simulink model "DynamicFFT_Ex2"  (R2024a)
settings: Solver=VariableStepAuto  StartTime=0.0  StopTime=2  RelTol=1e-3
model workspace (MAT data in the model file):
  frame_size = 512
  max_fft_size = 512
undefined symbols (not defined in the file): None, S, vsva2197, xcvc1902
libraries: matrix_library x2, aieDSP x1, dspobslib x1, dspsrcs4 x1, aieUtilities x1, vmcUtilities x1
settings Model: Creator=sdegala  LastModifiedBy=robg
settings ModelReferenceCC: EnableRefExpFcnMdlSchedulingChecks=on
settings RTWCC: GPUComputeCapability=3.5
settings ConfigComp: CovBoundaryAbsTol=1.0e-5

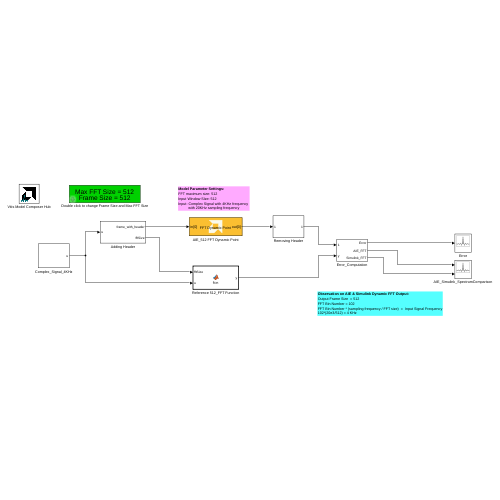
[thumbnail: Simulink's stored preview of the top-level diagram]
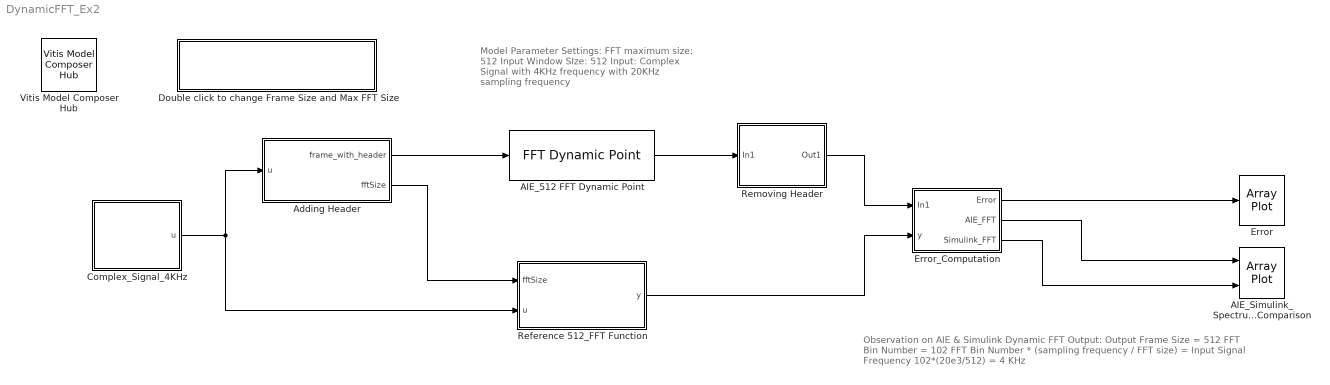
== system DynamicFFT_Ex2 ==
  note: Model Parameter Settings:
      | FFT maximum size: 512
      | Input Window SIze: 512
      | Input: Complex Signal with 4KHz frequency
      | with 20KHz sampling frequency
  note: Observation on AIE & Simulink Dynamic FFT Output:
      | Output Frame Size = 512
      | FFT Bin Number = 102
      | FFT Bin Number * (sampling frequency / FFT size) = Input Signal Frequency
      | 102*(20e3/512) = 4 KHz
  AIE_512 FFT Dynamic Point : aieDSP/FFT Dynamic Point  AIE_VARIANT=1  data_type=cfloat  data_out_type=cfloat  twiddle_type=cfloat  point_size=512  input_window_size=512  shift_val=0  rnd_mode=Round symmetrical to infinity  sat_mode=0-None  ssr=1  twiddle_mode=0  use_ssr_widget_kernels=off  casc_length=1  transform_fft_nifft=1  TP_API=0  TP_DYN_PT_SIZE=1  blockJsonConstraints=[]  blockJsonConstraintsInternal=[]  spec=vmc_dyn_pt_fft.json  SerializedMaskParamNames=[]  SerializedMaskParamValues=[]  SerializedMaskParamVisibilities=[]  block_type=FFT Dynamic Point  SerializedMaskParamDataypes=uint|typename|typename|typename|uint|uint|uint|uint|uint|uint|uint|uint|uint|uint|uint|uint  SerializedMaskParamEnumStrArr=0|0|0|0|0|0|0|Round to positive infinity,Round to negative infinity,Round symmetrical to infinity,Round symmetrical to zero,Round convergent to even,Round convergent to odd|0-None,1-Asymmetric,3-Symmetric|0|0|0|0|0|0|0  SerializedMaskParamEnumValArr=0|0|0|0|0|0|0|2,3,4,5,6,7|0,1,3|0|0|0|0|0|0|0  SerializedMaskParamVectorArr=0|0|0|0|0|0|0|0|0|0|0|0|0|0|0|0  SerializedMaskParamKeys=AIE_VARIANT|TT_DATA|TT_OUT_DATA|TT_TWIDDLE|TP_POINT_SIZE|TP_WINDOW_VSIZE|TP_SHIFT|TP_RND|TP_SAT|TP_PARALLEL_POWER|TP_TWIDDLE_MODE|TP_USE_WIDGETS|TP_CASC_LEN|TP_FFT_NIFFT|TP_API|TP_DYN_PT_SIZE
  AIE_Simulink_SpectrumComparison : ArrayPlot  NumInputPorts=2  WindowPosition=[5.000000,41.000000,1272.000000,651.000000,]  PlotType=Line  AxesScaling=Manual  YLimits=[-100,1100]  ShowLegend=on
  Adding Header : Subsystem
  Complex_Signal_4KHz : Subsystem
  Double click to change Frame Size and Max FFT Size : Subsystem  mask{max_fft_size=512, frame_size=512}
      mask prompts: max_fft_size "Max FFT Size"; frame_size "Frame Size"
      mask help: Set the FFT length
      mask TypeOptions max_fft_size: 128 | 256 | 512 | 1024 | 2048 | 4096
      mask Callback max_fft_size:
      | max_fft_size = str2double(get_param(gcb,'max_fft_size'));
      | hws = get_param(bdroot, 'modelworkspace');
      | hws.assignin('max_fft_size', max_fft_size);
      mask Callback frame_size:
      | frame_size = str2double(get_param(gcb,'frame_size'));
      | hws = get_param(bdroot, 'modelworkspace');
      | hws.assignin('frame_size', frame_size);
      mask Display:
      | max_fft_size = get_param(gcb,'max_fft_size');
      | frame_size = get_param(gcb,'frame_size');
      | 
      | disp(['\fontsize{18}Max FFT Size = ' max_fft_size newline 'Frame Size = ' frame_size], 'texmode', 'on');
  Error : ArrayPlot  WindowPosition=[432.000000,41.000000,845.000000,423.000000,]  PlotType=Line  AxesScaling=Manual  YLimits=[-5,5]  ShowLegend=on
  Error_Computation : Subsystem
  Reference 512_FFT Function : MATLAB Function  TreatAsAtomicUnit=on
  Removing Header : Subsystem
  Vitis Model Composer Hub : vmcUtilities/Vitis Model Composer Hub  Tag=genX  CodeGeneration=off  StartColumn=1  NumberOfColumns=1  TargetDirectory=./code  exportDesign=off  analyzeDesign=off  validateDesignOnHw=off  ExportType=AI Engines  IpVendor=xilinx.com  IpLibrary=hls  IpVersion=1.0  IpHWLanguage=Verilog  AieCompilerOptions={}  AieSimulatorOptions={}  CreateTestbench=off  TestbenchStackSize=10  RunRtlSim=off  RunCSim=off  RunAieSim=off  AieSimTimeout=50000  RunAieSimProfiling=off  LaunchVitisAnalyzer=off  PlotOutput=off  RunX86Sim=off  X86SimTimeout=10  GenHwImage=off  GenLibadfXo=off  GenHwValidationCode=off  PlatformType=Not Specified  HwSystemType=Baremetal  HwValidationTarget=hw  ProjDevice=xcvc1902-vsva2197-1LP-e-S  ProjDevicePart=xcvc1902-vsva2197-1LP-e-S  AIEType=AIE  SamplePeriod=-1  ClockFrequency=200  DataPathParallelism=1  xilinxfamily=versalaicore  part=xcvc1902  speed=-1LP-e-S  package=vsva2197  directory=./netlist  testbench=off  incr_netlist=off  synthesis_tool=Vivado  clock_wrapper=Clock Enables  dbl_ovrd=According to Block Masks  dcm_input_clock_period=10  sysclk_period=10  simulink_period=1  eval_field=0  LogFileName=''  NThreads=4
  wires:
  Complex_Signal_4KHz/1(u) -> Adding Header/1(u), Reference 512_FFT Function/2(u)
  Error_Computation/1(Error) -> Error/1
  Adding Header/2(fftSize) -> Reference 512_FFT Function/1(fftSize)
  AIE_512 FFT Dynamic Point/1 -> Removing Header/1(In1)
  Removing Header/1(Out1) -> Error_Computation/1(In1)
  Reference 512_FFT Function/1(y) -> Error_Computation/2(y)
  Adding Header/1(frame_with_header) -> AIE_512 FFT Dynamic Point/1
  Error_Computation/2(AIE_FFT) -> AIE_Simulink_SpectrumComparison/1
  Error_Computation/3(Simulink_FFT) -> AIE_Simulink_SpectrumComparison/2

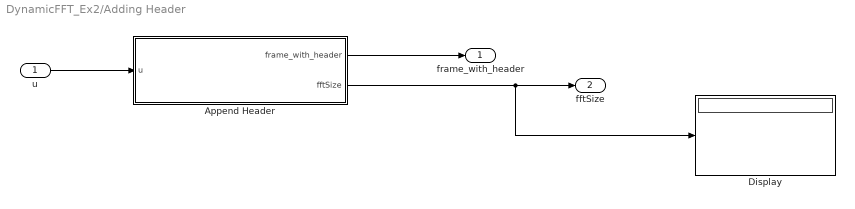
== system DynamicFFT_Ex2/Adding Header ==
  u : Inport
  Append Header : MATLAB Function  TreatAsAtomicUnit=on  mask{fftSizeInput=[128 512]}
      mask prompts: fftSizeInput "FFT Size"
      mask help:
      | This block appends a header to each incoming frame. The FFT Size parameter specifies an array of power of twos. These should be equal or smaller than the maximum size FFT specified for the Dynamic Point FFT block.
      |
      | As an example, if the FFT Size parameter is [128, 512, 1024] and the input size to this block is 1024, the Dynamic Point FFT block will take a 128 point FFT of the first 128 samples of the first input frame (discarding other samples), a 512 point FFT of the first 512 samples of the second input frame (discarding other samples), and a 1024 point FFT of the third input frame and all the subsequent input frames.
  Display : Display
  frame_with_header : Outport
  fftSize : Outport  Port=2
  wires:
  Append Header/2(fftSize) -> Display/1, fftSize/1
  Append Header/1(frame_with_header) -> frame_with_header/1
  u/1 -> Append Header/1(u)

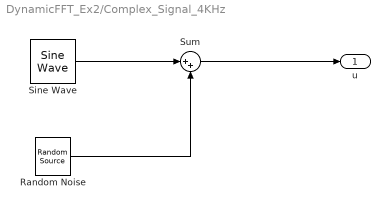
== system DynamicFFT_Ex2/Complex_Signal_4KHz ==
  Random Noise : dspobslib/Random Source  SrcType=Gaussian  NormMethod=Ziggurat  CltLength=12  MinVal=0  MaxVal=1  MeanVal=0  VarVal=1e-3  RepMode=Not repeatable  rawSeed=1  IsInherit=off  SampMode=Discrete  SampTime=1/20e3  SampFrame=512  DataType=Single  OutComplex=Real  OutputFrames=off
  Sine Wave : dspsrcs4/Sine Wave  Amplitude=1  Frequency=4e3  Phase=0  SampleMode=Discrete  OutComplex=Complex  CompMethod=Trigonometric fcn  TableSize=Speed  SampleTime=1/20e3  SamplesPerFrame=512  ResetState=Restart at time zero  OutputFrames=off  dataType=single  wordLen=16  udDataType=sfix(16)  fracBitsMode=Best precision  numFracBits=15  OutDataTypeStr=single  LastOutDataTypeStr=single
  Sum : Sum  Inputs=|++
  u : Outport
  wires:
  Sine Wave/1 -> Sum/1
  Sum/1 -> u/1
  Random Noise/1 -> Sum/2

== system DynamicFFT_Ex2/Double click to change Frame Size and Max FFT Size ==

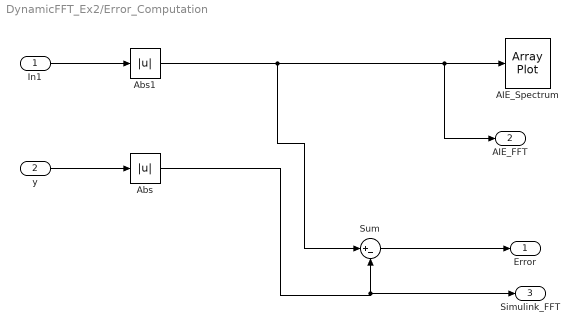
== system DynamicFFT_Ex2/Error_Computation ==
  In1 : Inport
  y : Inport  Port=2
  AIE_Spectrum : ArrayPlot  WindowPosition=[434.000000,41.000000,800.000000,500.000000,]  XDataMode=Custom  PlotType=Line  YLimits=[-48.2881,436.0459]  ShowLegend=on
  Abs : Abs  SaturateOnIntegerOverflow=off
  Abs1 : Abs  SaturateOnIntegerOverflow=off
  Sum : Sum  Inputs=|+-  AccumDataTypeStr=int32
  Error : Outport
  AIE_FFT : Outport  Port=2
  Simulink_FFT : Outport  Port=3
  wires:
  In1/1 -> Abs1/1
  y/1 -> Abs/1
  Abs1/1 -> Sum/1, AIE_FFT/1, AIE_Spectrum/1
  Sum/1 -> Error/1
  Abs/1 -> Simulink_FFT/1, Sum/2

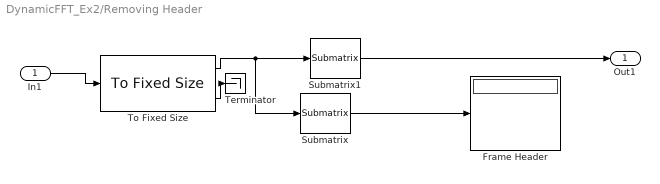
== system DynamicFFT_Ex2/Removing Header ==
  In1 : Inport
  Frame Header : Display
  Submatrix : matrix_library/Submatrix  RowSpan=Range of rows  RowStartMode=Index  RowStartIndex=1  RowEndMode=Index  RowEndIndex=4  ColSpan=One column  ColStartMode=First  ColStartIndex=1  ColEndMode=Last  ColEndIndex=1
  Submatrix1 : matrix_library/Submatrix  RowSpan=Range of rows  RowStartMode=Index  RowStartIndex=5  RowEndMode=Index  RowEndIndex=516  ColSpan=One column  ColStartMode=First  ColStartIndex=1  ColEndMode=Last  ColEndIndex=1
  Terminator : Terminator
  To Fixed Size : aieUtilities/To Fixed Size  Mode=Produce a valid output signal  OutputSize=516*1  CopyMethod=Buffer samples to form output  HasStatusOutput=on
  Out1 : Outport
  wires:
  To Fixed Size/2 -> Terminator/1
  Submatrix/1 -> Frame Header/1
  To Fixed Size/1 -> Submatrix/1, Submatrix1/1
  Submatrix1/1 -> Out1/1
  In1/1 -> To Fixed Size/1

== matlab function DynamicFFT_Ex2/Adding Header/Append Header ==
  data: u input; frame_with_header output; fftSizeInput parameter; fftSize output size=1
function [frame_with_header, fftSize] = fcn(u, fftSizeInput)

persistent inputFrameNum

if isempty(inputFrameNum)
    inputFrameNum = 1;    
end

headerValueSize = 4; % for int32 and Single data types.  
headerValue = zeros(headerValueSize,1);

% fftSize must be an array of power of twos that are smaller than input size

if any( fftSizeInput > length(u))
    error('fft sizes should be smaller or equal to the block input size.')
end

if ~all(log2(fftSizeInput) == round(log2(fftSizeInput)))
    error('fft sizes must be powers of two.')
end


% 0 for ifft, 1 for ifft
fftDir = 1; 

powerOf2 = log2(fftSizeInput(inputFrameNum)); 

% NOTE: For int16 the header is 8 samples and is in the form of [fftDir powerOf2 0 0 0 0 0 0];

if isa(u,'int32') || isa(u,'single')
    headerValue(:,1) = [fftDir powerOf2 0 0]';
else
    error('While Dynamic FFT block also supports input of type int16, this block only supports input data type of int32 or single.')
end

fftSize = single(fftSizeInput(inputFrameNum));

% Cap inputFrameNum
if inputFrameNum < length(fftSizeInput)
    inputFrameNum = inputFrameNum + 1;
end

frame_with_header = [headerValue(1:headerValueSize,1); u];

== matlab function DynamicFFT_Ex2/Reference 512_FFT Function ==
  data: fftSize input; u input; y output; frame_size parameter; max_fft_size parameter
function y = fcn(fftSize, u, frame_size, max_fft_size)

out = complex(zeros(frame_size,1));

for i = 0:frame_size/max_fft_size-1
    frame_fft = fft(double(u(i*max_fft_size+1:(i+1)*max_fft_size)),fftSize);
    out(i*max_fft_size+1:(i+1)*max_fft_size) = [frame_fft; zeros(max_fft_size - fftSize,1)];
end

y = single(out(1:frame_size));
